simulink library "Golf_Components_Lib"  (R2018a)
settings: Solver=ode45  StartTime=0.0  StopTime=10.0  RelTol=1e-3  EnableMultiTasking=on
undefined symbols (not defined in the file): Plane_Data_Ring, X, Y, Z
libraries: sm_lib x63, Contact_Forces_Lib x21, nesl_utility x4
(part 1 of 3)
Description:
  | Copyright 2015-2019 The MathWorks, Inc.
settings Model: Creator=smiller  LastModifiedBy=smiller
settings DataIOCC: LimitDataPoints=on  SaveFormat=Array  SignalLoggingSaveFormat=ModelDataLogs
settings OptimizationCC: ExpressionDepthLimit=2147483647  LifeSpan=inf
settings DebuggingCC: UnderspecifiedInitializationDetection=Classic  MergeDetectMultiDrivingBlocksExec=none  SolverPrmCheckMsg=warning  FcnCallInpInsideContextMsg=warning  AllowSymbolicDim=off  StateNameClashWarn=warning  SFUnexpectedBacktrackingDiag=warning  SFNoUnconditionalDefaultTransitionDiag=warning  SFExecutionAtInitializationDiag=none
settings HardwareCC: ProdBitPerPointer=32  ProdBitPerSizeT=32  ProdBitPerPtrDiffT=32  ProdLargestAtomicFloat=None  ProdIntDivRoundTo=Undefined  ProdEndianess=Unspecified  ProdWordSize=32  ProdHWDeviceType=32-bit Generic
settings ModelReferenceCC: PropagateSignalLabelsOutOfModel=off
settings CodeAppCC: StateflowObjectComments=on
settings GRTTargetCC: TargetLangStandard=C89/C90 (ANSI)  GeneratePreprocessorConditionals=Disable all
settings ConfigComp: CovMetricSettings=dw  CovHtmlReporting=on  CovSaveCumulativeToWorkspaceVar=on  CovSaveSingleToWorkspaceVar=on  CovExternalEMLEnable=off  CovSFcnEnable=off

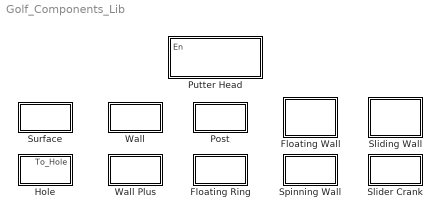
== system Golf_Components_Lib ==
  Floating Ring : Subsystem  mask(Floating Ring, 2D Contacts){extr_xy_data=Plane_Data_Ring(0.5,0.4), offset=[5.7 0 0], height=0.0853, diameter=0.5, extr1_friction=0.3, ball_radius=0.04267, contact_k=1e5, contact_b=10, low_pass_filt_const=1e-4}
      mask prompts: extr_xy_data "Extrusion XY Data (m)"; offset "Offset (x,y,z)"; diameter "Outer Diameter (m)"; extr1_friction "Friction (N/(m/s))"; ball_radius "Ball Radius (m)"; contact_k "Contact Stiffness"; contact_b "Contact Damping"; low_pass_filt_const "Low Pass Filter Constant"
      mask help:
      | Parameterized ring with integrated contact forces that will repel a circle.  The ring can translate only within the XY plane.
      |
      | The port must be connected to a frame located at the center of a circle.  The Ref Frame should be connected to the World Frame.
  Floating Wall : Subsystem  mask(Floating Wall with Round Ends, 2D Contacts){length=1.8, angle=0, offset=[5 0 0], height=0.0853, width=0.1, wall_friction=0.3, wall_rot_friction=0.1, ball_radius=0.04267, contact_k=1e5, contact_b=10, low_pass_filt_const=1e-4}
      mask prompts: length "Length (m)"; angle "Angle (deg)"; offset "Offset (x,y,z)"; wall_friction "Wall Sliding Friction(N/(m/s))"; wall_rot_friction "Wall Spinning Friction(N*m/(rad/s))"; ball_radius "Ball Radius (m)"; contact_k "Contact Stiffness"; contact_b "Contact Damping"; low_pass_filt_const "Low Pass Filter Constant"
      mask help:
      | Parameterized wall section with round ends with integrated contact forces that will repel a circle.  The wall can translate and rotate within the XY-plane.
      |
      | The Ball port must be connected to a frame located at the center of a circle. The Ref port should be connected to the World Frame. The C1 and C2 ports are connected to frames at the centers of the circles at either end of the wall.  Connecting these to Circle-to-Plane forces will enable the wall to bounce off of other walls.
  Hole : Subsystem  mask(Golf Course Hole, with Attractor Force){hole_offset=[5.5  0   -0.05], hole_radius=0.1079, hole_height=0.0505, hole_stiffness=-1e4, hole_damping=10, hole_deadzone=0.6667}
      mask prompts: hole_offset "Hole Location (x,y,z)"; hole_radius "Hole Radius (m)"; hole_height "Hole Height(m)"; hole_stiffness "Hole Attraction Stiffness"; hole_damping "Hole Attraction Damping"; hole_deadzone "Hole Deadzone (m)/Hole Radius (m)"
      mask help: Creates a hole for the golf course. The circle-to-circle attraction force will draw the ball into the hole if it gets close enough. The deadzone at the center of the hole is to reduce oscillations when the ball arrives. Outputs are the distance from the ball to the hole (x, y, r, and theta).
      mask DialogControl ParameterTabVar0 Prompt: Location
      mask DialogControl ParameterTabVar01 Prompt: Dimensions
      mask DialogControl ParameterTabVar012 Prompt: Contact
  Post : Subsystem  mask(Round Obstacle, 2D Contacts){width=1.2, height=0.0853, offset=[2.2 -0.25 0], ball_radius=0.04267, contact_k=1e5, contact_b=10, low_pass_filt_const=1e-4}
      mask prompts: width "Diameter (m)"; height "Height (m)"; offset "Offset (x,y,z)"; ball_radius "Ball Radius (m)"; contact_k "Contact Stiffness"; contact_b "Contact Damping"; low_pass_filt_const "Low Pass Filter Constant"
      mask help:
      | Parameterized round obstacle with integrated contact forces that will repel a circle.
      |
      | The Ball port must be connected to a frame located at the center of a circle.  The Ref port should be connected to a World Frame.
  Putter Head : Subsystem  mask(Wall with Round Ends, 2D Contact Forces){length=0.1270, height=0.03, width=0.05, ball_radius=0.04267, contact_k=1e5, contact_b=10, low_pass_filt_const=1e-4}
      mask prompts: length "Length (m)"; ball_radius "Ball Radius (m)"; contact_k "Contact Stiffness"; contact_b "Contact Damping"; low_pass_filt_const "Low Pass Filter Constant"
      mask help: Parameterized wall section with round ends with integrated contact forces that will repel a circle. The port must be connected to a frame located at the center of a circle.
      mask Display:
      | image(imread('Putter_Head_IMAGE.jpg'));
      | port_label('input',1,'En');
      | port_label('LConn',1,'CG');
      | port_label('RConn',1,'Ball');
  Slider Crank : Subsystem  mask(Slider Crank){initial_crank_spd=1, initial_crank_ang=0, rod_pin_radius=0.01, rod_pin_length=0.15, rod_pin_z_offset=-0.05, rod_dims=[0.025 0.75 0.015], rod_z_offset=-0.05, crank_pin_radius=0.01, crank_pin_length=0.05, crank_radius=0.25, crank_length=0.05, crank_z_offset=-0.05, density=1000}
      mask prompts: initial_crank_spd "Initial Crank Speed (rad/s)"; initial_crank_ang "Initial Crank Angle (deg)"; rod_pin_radius "Rod Pin Radius (m)"; rod_pin_length "Rod Pin Length (m)"; rod_pin_z_offset "Rod Pin Z Offset (m)"; rod_dims "Rod Dimensions (m)"; rod_z_offset "Rod Z Offset (m)"; crank_pin_radius "Crank Pin Radius (m)"; crank_pin_length "Crank Pin Length (m)"; crank_radius "Crank Radius (m)"; crank_length "Crank_Length (m)"; crank_z_offset "Crank Z Offset (m)"; density "Part Density (kg/m^3)"
      mask help:
      | Crank, sliding rod, and pin for connection to a slider.
      |
      | FRodPin should be connected to the part representing the slider.  FCrankCG should be attached to the World Frame at the same location as FRodPin.  Mechanism is parameterized relative to the slider pin location.
  Sliding Wall : Subsystem  mask(Sliding Wall with Round Ends, 2D Contacts){length=2, angle=0, offset=[1.5 -0.5 0], height=0.0853, width=0.1, wall_density=1000, ball_radius=0.0427, contact_k=1e5, contact_b=10, low_pass_filt_const=1e-4}
      mask prompts: length "Length (m)"; angle "Angle (deg)"; offset "Offset (x,y,z)"; wall_density "Wall Density (kg/m3)"; ball_radius "Ball Radius (m)"; contact_k "Contact Stiffness"; contact_b "Contact Damping"; low_pass_filt_const "Low Pass Filter Constant"
      mask help:
      | Parameterized wall section with round ends with integrated contact forces that will repel a circle.  This wall can slide along the Y axis only.
      |
      | The port must be connected to a frame located at the center of a circle. The Ref port should be connected to the World Frame.
      |
      | The WRf port is attached to the same part as Ref, and located at the center of the Offset position of the wall.  The Wall port is attached to the Wall CG, and is where the actuation for sliding can be attached.
  Spinning Wall : Subsystem  mask(Spinning Wall with Round Ends, 2D Contacts){length=1.8, angle=0, offset=[4 0 0], ang_spd=1, height=0.0853, width=0.1, wall_density=1000, ball_radius=0.0427, contact_k=1e5, contact_b=10, low_pass_filt_const=1e-4}
      mask prompts: length "Length (m)"; angle "Angle (deg)"; offset "Offset (x,y,z)"; ang_spd "Initial Speed (rad/s)"; wall_density "Wall Density (kg/m3)"; ball_radius "Ball Radius (m)"; contact_k "Contact Stiffness"; contact_b "Contact Damping"; low_pass_filt_const "Low Pass Filter Constant"
      mask help:
      | Parameterized wall section with round ends with integrated contact forces that will repel a circle.  This wall can rotate only within the XY plane.
      |
      | The port must be connected to a frame located at the center of a circle. The Ref port should be connected to the World Frame. Additional wall sections that will also rotate may be connected to the CG port.
  Surface : Subsystem  mask(Square Surface Patch for Golf Course){width=2, length=6, offset=[3 0 -0.05], height=0.05}
      mask prompts: width "Surface Width (m)"; length "Surface Length (m)"; offset "Surface Offset (m)"; height "Surface Thickness(m)"
      mask help: Creates a square surface patch for golf course. All parameters are relative to the frame that is connected to the port.
  Wall : Subsystem  mask(Wall with Round Ends, 2D Contacts){length=2, angle=0, offset=[6 0 0], height=0.0853, width=0.1, wall_density=1000, ball_radius=0.0427, contact_k=1e5, contact_b=10, low_pass_filt_const=1e-4}
      mask prompts: length "Length (m)"; angle "Angle (deg)"; offset "Offset (x,y,z)"; wall_density "Wall Density (kg/m3)"; ball_radius "Ball Radius (m)"; contact_k "Contact Stiffness"; contact_b "Contact Damping"; low_pass_filt_const "Low Pass Filter Constant"
      mask help: Parameterized wall section with round ends with integrated contact forces that will repel a circle. The Ball port must be connected to a frame located at the center of a circle. The Ref port should be connected to a World Frame
  Wall Plus : Subsystem  mask(Wall with Round Ends, 2D Contacts, Port at CG){length=2, angle=0, offset=[6 0 0], height=0.0853, width=0.1, ball_radius=0.04267, contact_k=1e5, contact_b=10, low_pass_filt_const=1e-4}
      mask prompts: length "Length (m)"; angle "Angle (deg)"; offset "Offset (x,y,z)"; ball_radius "Ball Radius (m)"; contact_k "Contact Stiffness"; contact_b "Contact Damping"; low_pass_filt_const "Low Pass Filter Constant"
      mask help: Parameterized wall section with round ends with integrated contact forces that will repel a circle. The Ball port must be connected to a frame located at the center of a circle. The Ref port should be connected to the World Frame. The Pla port can be used for addding additional contact forces.

== system Golf_Components_Lib/Floating Ring ==
  2-D Contact Force Circle to Circle1 : Contact_Forces_Lib/2D/Circle to Circle Force  cirB_rad=diameter/2  cirF_rad=ball_radius  active_angle=[-180 180]  force_law=Linear  k_contact=contact_k  b_contact=contact_b  pen_full_damp_F=1e-4  pen_exponent=1  custom_param_1=1  custom_param_2=1  friction_law=None  mu_kinetic=0.5  mu_static=0.7  v_thr=0.001  vis_on=off  vis_opc_en=0  vis_len_cirBz=0.1  vis_len_cirBx=0.005  vis_len_cirFz=0.1  vis_len_cirFx=0.005  vis_clr=[0.9 0.2 0.2]  vis_opc=0.7
      settings: SourceProductName=Simscape Multibody Contact Forces Library
  Offset and Angle : sm_lib/Frames and Transforms/Rigid Transform  TranslationMethod=Cartesian  TranslationStandardOffset=0  TranslationLengthUnit=m  TranslationStandardAxis=+Y  TranslationCartesianOffset=offset  TranslationROffset=0  TranslationROffsetUnits=m  TranslationZOffset=0  TranslationZOffsetUnits=m  TranslationThetaOffset=0  TranslationThetaOffsetUnits=deg  RotationMethod=None  RotationAngleUnits=deg  RotationStandardAxis=+Z  RotationAngle=0  RotationArbitraryAxis=[0 0 1]  FollAlignAxisA=+X  BaseAlignAxisA=+Y  FollAlignAxisB=+Y  BaseAlignAxisB=+Z  RotationSequenceAxes=FollowerAxes  RotationSequence=XYX  RotationSequenceAngles=[0 0 0]  RotationSequenceAnglesUnits=deg  RotationMatrix=[1 0 0; 0 1 0; 0 0 1]
  Rectangular Joint : sm_lib/Joints/Rectangular Joint  SenseConstraintForce=off  SenseConstraintForceX=off  SenseConstraintForceY=off  SenseConstraintForceZ=off  SenseConstraintTorque=off  SenseConstraintTorqueX=off  SenseConstraintTorqueY=off  SenseConstraintTorqueZ=off  SenseTotalForce=off  SenseTotalForceX=off  SenseTotalForceY=off  SenseTotalForceZ=off  SenseTotalTorque=off  SenseTotalTorqueX=off  SenseTotalTorqueY=off  SenseTotalTorqueZ=off  CompositeWrenchDir=FollowerOnBase  CompositeWrenchFrame=BaseFrame  PxEquilibriumPosition=0  PxEquilibriumPositionUnits=m  PxSpringStiffness=0  PxSpringStiffnessUnits=N/m  PxDampingCoefficient=extr1_friction  PxDampingCoefficientUnits=N/(m/s)  PxTorqueActuationMode=NoTorque  PxMotionActuationMode=ComputedMotion  PxSensePosition=off  PxSenseVelocity=off  PxSenseAcceleration=off  PxSenseTorqueForce=off  PxPositionTargetSpecify=off  PxPositionTargetPriority=High  PxPositionTargetValue=0  PxPositionTargetValueUnits=m  PxVelocityTargetSpecify=off  PxVelocityTargetPriority=High  PxVelocityTargetValue=0  PxVelocityTargetValueUnits=m/s  PyEquilibriumPosition=0  PyEquilibriumPositionUnits=m  PySpringStiffness=0  PySpringStiffnessUnits=N/m  PyDampingCoefficient=extr1_friction  PyDampingCoefficientUnits=N/(m/s)  PyTorqueActuationMode=NoTorque  PyMotionActuationMode=ComputedMotion  PySensePosition=off  PySenseVelocity=off  PySenseAcceleration=off  PySenseTorqueForce=off  PyPositionTargetSpecify=off  PyPositionTargetPriority=High  PyPositionTargetValue=0  PyPositionTargetValueUnits=m  PyVelocityTargetSpecify=off  PyVelocityTargetPriority=High  PyVelocityTargetValue=0  PyVelocityTargetValueUnits=m/s
      settings: SourceProductName=Simscape Multibody
  Ring : sm_lib/Body Elements/Solid  InertiaType=CalculateFromGeometry  Mass=1  MassUnits=kg  CenterOfMass=[0 0 0]  CenterOfMassUnits=m  MomentsOfInertia=[1 1 1]  MomentsOfInertiaUnits=kg*m^2  ProductsOfInertia=[0 0 0]  ProductsOfInertiaUnits=kg*m^2  DensityBased=on  Density=Mini_Golf_Param.Hole_7.Wall_Obst1.Density  DensityUnits=kg/(m^3)  DoExposeReferenceFrame=on  SerializedFrames=<Frames/>  GraphicType=FromGeometry  MarkerShape=Sphere  MarkerSize=10  MarkerSizeUnits=m  GraphicVisPropType=SimpleVisualProperties  GraphicDiffuseColor=[0.5 0.5 0.5]  GraphicSpecularColor=[0.5 0.5 0.5 1.0]  GraphicAmbientColor=[0.15 0.15 0.15 1.0]  GraphicEmissiveColor=[0.0 0.0 0.0 1.0]  GraphicShininess=75  GraphicOpacity=1.0  GeometryShape=GeneralExtrusion  RectangleSize=[1 1]  RectangleSizeUnits=m  BrickDimensions=[1 1 1]  BrickDimensionUnits=m  CylinderRadius=1  CylinderRadiusUnits=m  CylinderLength=1  CylinderLengthUnits=m  SphereRadius=1  SphereRadiusUnits=m  EllipsoidRadii=[1 1 1]  EllipsoidRadiiUnits=m  ExtrusionCrossSection=extr_xy_data  ExtrusionCrossSectionUnits=m  ExtrusionLength=height  ExtrusionLengthUnits=m  PolygonNumSides=3  PolygonOuterRadius=1  PolygonOuterRadiusUnits=m  ExtGeomFileType=STL  ExtGeomFileUnits=m  RevolutionCrossSection=[1 1; 1 -1; 2 -1; 2 1]  RevolutionCrossSectionUnits=m  RevolutionExtent=Full  RevolutionAngle=180  RevolutionAngleUnits=deg
  Terminator : Terminator
  Ball : PMIOPort  Side=Right
  Ref : PMIOPort  Port=2  Side=Left
  CG : PMIOPort  Port=3  Side=Left
  wires:
  2-D Contact Force Circle to Circle1/1 -> Terminator/1
  connections:
  Offset and Angle/LConn1 -- Ref/RConn1
  Offset and Angle/RConn1 -- Rectangular Joint/RConn1
  2-D Contact Force Circle to Circle1/RConn1 -- CG/RConn1 -- Rectangular Joint/LConn1 -- Ring/RConn1
  2-D Contact Force Circle to Circle1/LConn1 -- Ball/RConn1

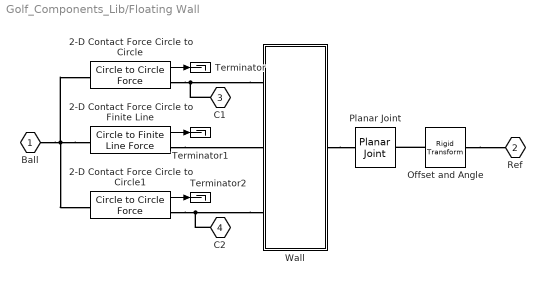
== system Golf_Components_Lib/Floating Wall ==
  2-D Contact Force Circle to Circle : Contact_Forces_Lib/2D/Circle to Circle Force  cirB_rad=width/2  cirF_rad=ball_radius  active_angle=[-180 180]  force_law=Linear  k_contact=contact_k  b_contact=contact_b  pen_full_damp_F=1e-4  pen_exponent=1  custom_param_1=1  custom_param_2=1  friction_law=None  mu_kinetic=0.5  mu_static=0.7  v_thr=0.001  vis_on=off  vis_opc_en=0  vis_len_cirBz=0.1  vis_len_cirBx=0.005  vis_len_cirFz=0.1  vis_len_cirFx=0.005  vis_clr=[0.9 0.2 0.2]  vis_opc=0.7
      settings: SourceProductName=Simscape Multibody Contact Forces Library
  2-D Contact Force Circle to Circle1 : Contact_Forces_Lib/2D/Circle to Circle Force  cirB_rad=width/2  cirF_rad=ball_radius  active_angle=[-180 180]  force_law=Linear  k_contact=contact_k  b_contact=contact_b  pen_full_damp_F=1e-4  pen_exponent=1  custom_param_1=1  custom_param_2=1  friction_law=None  mu_kinetic=0.5  mu_static=0.7  v_thr=0.001  vis_on=off  vis_opc_en=0  vis_len_cirBz=0.1  vis_len_cirBx=0.005  vis_len_cirFz=0.1  vis_len_cirFx=0.005  vis_clr=[0.9 0.2 0.2]  vis_opc=0.7
      settings: SourceProductName=Simscape Multibody Contact Forces Library
  2-D Contact Force Circle to Finite Line : Contact_Forces_Lib/2D/Circle to Finite Line Force  circle_rad=ball_radius  line_depth=width/2  line_length=length  force_law=Linear  k_contact=contact_k  b_contact=contact_b  pen_full_damp_F=1e-4  pen_exponent=1  custom_param_1=1  custom_param_2=1  friction_law=None  mu_kinetic=0.5  mu_static=0.7  v_thr=0.001  vis_on=off  vis_opc_en=0  vis_len_linBz=0.1  vis_len_linBx=0.005  vis_len_cirFz=0.1  vis_len_cirFx=0.005  vis_clr=[0.9 0.2 0.2]  vis_opc=0.7
      settings: SourceProductName=Simscape Multibody Contact Forces Library
  Offset and Angle : sm_lib/Frames and Transforms/Rigid Transform  TranslationMethod=Cartesian  TranslationStandardOffset=length/2  TranslationLengthUnit=m  TranslationStandardAxis=+Y  TranslationCartesianOffset=offset  TranslationROffset=0  TranslationROffsetUnits=m  TranslationZOffset=0  TranslationZOffsetUnits=m  TranslationThetaOffset=0  TranslationThetaOffsetUnits=deg  RotationMethod=StandardAxis  RotationAngleUnits=deg  RotationStandardAxis=+Z  RotationAngle=angle  RotationArbitraryAxis=[0 0 1]  FollAlignAxisA=+X  BaseAlignAxisA=+Y  FollAlignAxisB=+Y  BaseAlignAxisB=+Z  RotationSequenceAxes=FollowerAxes  RotationSequence=XYX  RotationSequenceAngles=[0 0 0]  RotationSequenceAnglesUnits=deg  RotationMatrix=[1 0 0; 0 1 0; 0 0 1]
  Planar Joint : sm_lib/Joints/Planar Joint  SenseConstraintForce=off  SenseConstraintForceX=off  SenseConstraintForceY=off  SenseConstraintForceZ=off  SenseConstraintTorque=off  SenseConstraintTorqueX=off  SenseConstraintTorqueY=off  SenseConstraintTorqueZ=off  SenseTotalForce=off  SenseTotalForceX=off  SenseTotalForceY=off  SenseTotalForceZ=off  SenseTotalTorque=off  SenseTotalTorqueX=off  SenseTotalTorqueY=off  SenseTotalTorqueZ=off  CompositeWrenchDir=FollowerOnBase  CompositeWrenchFrame=BaseFrame  PxEquilibriumPosition=0  PxEquilibriumPositionUnits=m  PxSpringStiffness=0  PxSpringStiffnessUnits=N/m  PxDampingCoefficient=wall_friction  PxDampingCoefficientUnits=N/(m/s)  PxTorqueActuationMode=NoTorque  PxMotionActuationMode=ComputedMotion  PxSensePosition=off  PxSenseVelocity=off  PxSenseAcceleration=off  PxSenseTorqueForce=off  PxPositionTargetSpecify=off  PxPositionTargetPriority=High  PxPositionTargetValue=0  PxPositionTargetValueUnits=m  PxVelocityTargetSpecify=off  PxVelocityTargetPriority=High  PxVelocityTargetValue=0  PxVelocityTargetValueUnits=m/s  PyEquilibriumPosition=0  PyEquilibriumPositionUnits=m  PySpringStiffness=0  PySpringStiffnessUnits=N/m  PyDampingCoefficient=wall_friction  PyDampingCoefficientUnits=N/(m/s)  PyTorqueActuationMode=NoTorque  PyMotionActuationMode=ComputedMotion  PySensePosition=off  PySenseVelocity=off  PySenseAcceleration=off  PySenseTorqueForce=off  PyPositionTargetSpecify=off  PyPositionTargetPriority=High  PyPositionTargetValue=0  PyPositionTargetValueUnits=m  PyVelocityTargetSpecify=off  PyVelocityTargetPriority=High  PyVelocityTargetValue=0  PyVelocityTargetValueUnits=m/s  RzEquilibriumPosition=0  RzEquilibriumPositionUnits=rad  RzSpringStiffness=0  RzSpringStiffnessUnits=N*m/rad  RzDampingCoefficient=wall_rot_friction  RzDampingCoefficientUnits=N*m/(rad/s)  RzTorqueActuationMode=NoTorque  RzMotionActuationMode=ComputedMotion  RzSensePosition=off  RzSenseVelocity=off  RzSenseAcceleration=off  RzSenseTorqueForce=off  RzPositionTargetSpecify=off  RzPositionTargetPriority=High  RzPositionTargetValue=0  RzPositionTargetValueUnits=rad  RzVelocityTargetSpecify=off  RzVelocityTargetPriority=High  RzVelocityTargetValue=0  RzVelocityTargetValueUnits=rad/s
  Terminator : Terminator
  Terminator1 : Terminator
  Terminator2 : Terminator
  Wall : Subsystem
  Ball : PMIOPort  Side=Right
  Ref : PMIOPort  Port=2  Side=Left
  C1 : PMIOPort  Port=3  Side=Left
  C2 : PMIOPort  Port=4  Side=Left
  wires:
  2-D Contact Force Circle to Circle/1 -> Terminator/1
  2-D Contact Force Circle to Finite Line/1 -> Terminator1/1
  2-D Contact Force Circle to Circle1/1 -> Terminator2/1
  connections:
  2-D Contact Force Circle to Finite Line/LConn1 -- 2-D Contact Force Circle to Circle1/LConn1 -- Ball/RConn1 -- 2-D Contact Force Circle to Circle/LConn1
  Offset and Angle/RConn1 -- Planar Joint/LConn1
  Offset and Angle/LConn1 -- Ref/RConn1
  Wall/RConn1 -- C1/RConn1 -- 2-D Contact Force Circle to Circle/RConn1
  2-D Contact Force Circle to Finite Line/RConn1 -- Wall/RConn2
  Wall/LConn1 -- Planar Joint/RConn1
  Wall/RConn3 -- C2/RConn1 -- 2-D Contact Force Circle to Circle1/RConn1

== system Golf_Components_Lib/Hole ==
  2-D Attraction Force Circle to Hole : Contact_Forces_Lib/2D/Circle to Hole Force  k_contact=hole_stiffness  b_contact=hole_damping  max_frame_sep=hole_radius  active_angle=[-180 180]  h_deadzone=hole_deadzone
      settings: SourceProductName=Simscape Multibody Contact Forces Library
  Hole : sm_lib/Body Elements/Solid  InertiaType=CalculateFromGeometry  Mass=1  MassUnits=kg  CenterOfMass=[0 0 0]  CenterOfMassUnits=m  MomentsOfInertia=[1 1 1]  MomentsOfInertiaUnits=kg*m^2  ProductsOfInertia=[0 0 0]  ProductsOfInertiaUnits=kg*m^2  DensityBased=on  Density=100  DensityUnits=kg/(m^3)  DoExposeReferenceFrame=on  SerializedFrames=<Frames/>  GraphicType=FromGeometry  MarkerShape=Sphere  MarkerSize=10  MarkerSizeUnits=m  GraphicVisPropType=SimpleVisualProperties  GraphicDiffuseColor=[0.0 0.0 0.0]  GraphicSpecularColor=[0.5 0.5 0.5 1.0]  GraphicAmbientColor=[0.15 0.15 0.15 1.0]  GraphicEmissiveColor=[0.0 0.0 0.0 1.0]  GraphicShininess=75  GraphicOpacity=1.0  GeometryShape=Cylinder  RectangleSize=[1 1]  RectangleSizeUnits=m  BrickDimensions=[1 1 1]  BrickDimensionUnits=m  CylinderRadius=hole_radius  CylinderRadiusUnits=m  CylinderLength=hole_height  CylinderLengthUnits=m  SphereRadius=1  SphereRadiusUnits=m  EllipsoidRadii=[1 1 1]  EllipsoidRadiiUnits=m  ExtrusionCrossSection=[1 1; -1 1; -1 -1; 1 -1]  ExtrusionCrossSectionUnits=m  ExtrusionLength=1  ExtrusionLengthUnits=m  PolygonNumSides=3  PolygonOuterRadius=1  PolygonOuterRadiusUnits=m  ExtGeomFileType=STL  ExtGeomFileUnits=m  RevolutionCrossSection=[1 1; 1 -1; 2 -1; 2 1]  RevolutionCrossSectionUnits=m  RevolutionExtent=Full  RevolutionAngle=180  RevolutionAngleUnits=deg
  Rigid Transform : sm_lib/Frames and Transforms/Rigid Transform  TranslationMethod=Cartesian  TranslationStandardOffset=0  TranslationLengthUnit=m  TranslationStandardAxis=+Z  TranslationCartesianOffset=hole_offset  TranslationROffset=0  TranslationROffsetUnits=m  TranslationZOffset=0  TranslationZOffsetUnits=m  TranslationThetaOffset=0  TranslationThetaOffsetUnits=deg  RotationMethod=None  RotationAngleUnits=deg  RotationStandardAxis=+Z  RotationAngle=0  RotationArbitraryAxis=[0 0 1]  FollAlignAxisA=+X  BaseAlignAxisA=+Y  FollAlignAxisB=+Y  BaseAlignAxisB=+Z  RotationSequenceAxes=FollowerAxes  RotationSequence=XYX  RotationSequenceAngles=[0 0 0]  RotationSequenceAnglesUnits=deg  RotationMatrix=[1 0 0; 0 1 0; 0 0 1]
  Sensing : Subsystem
  Terminator : Terminator
  Ball : PMIOPort  Side=Left
  Ref : PMIOPort  Port=2  Side=Right
  To_Hole : Outport
  wires:
  Sensing/1(To_Hole) -> To_Hole/1
  2-D Attraction Force Circle to Hole/1 -> Terminator/1
  connections:
  Rigid Transform/LConn1 -- Ref/RConn1
  Hole/RConn1 -- Rigid Transform/RConn1 -- Sensing/RConn1 -- 2-D Attraction Force Circle to Hole/RConn1
  Sensing/LConn1 -- Ball/RConn1 -- 2-D Attraction Force Circle to Hole/LConn1

== system Golf_Components_Lib/Post ==
  2-D Contact Force Circle to Circle : Contact_Forces_Lib/2D/Circle to Circle Force  cirB_rad=width/2  cirF_rad=ball_radius  active_angle=[-180 180]  force_law=Linear  k_contact=contact_k  b_contact=contact_b  pen_full_damp_F=1e-4  pen_exponent=1  custom_param_1=1  custom_param_2=1  friction_law=None  mu_kinetic=0.5  mu_static=0.7  v_thr=0.001  vis_on=off  vis_opc_en=0  vis_len_cirBz=0.1  vis_len_cirBx=0.005  vis_len_cirFz=0.1  vis_len_cirFx=0.005  vis_clr=[0.9 0.2 0.2]  vis_opc=0.7
      settings: SourceProductName=Simscape Multibody Contact Forces Library
  Offset and Angle : sm_lib/Frames and Transforms/Rigid Transform  TranslationMethod=Cartesian  TranslationStandardOffset=0  TranslationLengthUnit=m  TranslationStandardAxis=+Y  TranslationCartesianOffset=offset  TranslationROffset=0  TranslationROffsetUnits=m  TranslationZOffset=0  TranslationZOffsetUnits=m  TranslationThetaOffset=0  TranslationThetaOffsetUnits=deg  RotationMethod=None  RotationAngleUnits=deg  RotationStandardAxis=+Z  RotationAngle=0  RotationArbitraryAxis=[0 0 1]  FollAlignAxisA=+X  BaseAlignAxisA=+Y  FollAlignAxisB=+Y  BaseAlignAxisB=+Z  RotationSequenceAxes=FollowerAxes  RotationSequence=XYX  RotationSequenceAngles=[0 0 0]  RotationSequenceAnglesUnits=deg  RotationMatrix=[1 0 0; 0 1 0; 0 0 1]
  Post : sm_lib/Body Elements/Solid  InertiaType=CalculateFromGeometry  Mass=1  MassUnits=kg  CenterOfMass=[0 0 0]  CenterOfMassUnits=m  MomentsOfInertia=[1 1 1]  MomentsOfInertiaUnits=kg*m^2  ProductsOfInertia=[0 0 0]  ProductsOfInertiaUnits=kg*m^2  DensityBased=on  Density=1  DensityUnits=kg/(m^3)  DoExposeReferenceFrame=on  SerializedFrames=<Frames/>  GraphicType=FromGeometry  MarkerShape=Sphere  MarkerSize=10  MarkerSizeUnits=m  GraphicVisPropType=SimpleVisualProperties  GraphicDiffuseColor=[0.5 0.5 0.5]  GraphicSpecularColor=[0.5 0.5 0.5 1.0]  GraphicAmbientColor=[0.15 0.15 0.15 1.0]  GraphicEmissiveColor=[0.0 0.0 0.0 1.0]  GraphicShininess=75  GraphicOpacity=1.0  GeometryShape=Cylinder  RectangleSize=[1 1]  RectangleSizeUnits=m  BrickDimensions=[1 1 1]  BrickDimensionUnits=m  CylinderRadius=width/2  CylinderRadiusUnits=m  CylinderLength=height  CylinderLengthUnits=m  SphereRadius=1  SphereRadiusUnits=m  EllipsoidRadii=[1 1 1]  EllipsoidRadiiUnits=m  ExtrusionCrossSection=[1 1; -1 1; -1 -1; 1 -1]  ExtrusionCrossSectionUnits=m  ExtrusionLength=1  ExtrusionLengthUnits=m  PolygonNumSides=3  PolygonOuterRadius=1  PolygonOuterRadiusUnits=m  ExtGeomFileType=STL  ExtGeomFileUnits=m  RevolutionCrossSection=[1 1; 1 -1; 2 -1; 2 1]  RevolutionCrossSectionUnits=m  RevolutionExtent=Full  RevolutionAngle=180  RevolutionAngleUnits=deg
  Terminator : Terminator
  Ball : PMIOPort  Side=Right
  Ref : PMIOPort  Port=2  Side=Left
  wires:
  2-D Contact Force Circle to Circle/1 -> Terminator/1
  connections:
  Ball/RConn1 -- 2-D Contact Force Circle to Circle/LConn1
  Offset and Angle/RConn1 -- 2-D Contact Force Circle to Circle/RConn1 -- Post/RConn1
  Offset and Angle/LConn1 -- Ref/RConn1

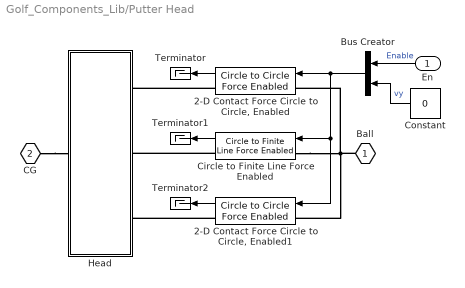
== system Golf_Components_Lib/Putter Head ==
  En : Inport
  "2-D Contact Force Circle to Circle, Enabled" : Contact_Forces_Lib/2D/Circle to Circle Force Enabled  cirB_rad=width/2  cirF_rad=ball_radius  active_angle=[-180 180]  force_law=Linear  k_contact=contact_k  b_contact=contact_b  pen_full_damp_F=1e-4  pen_exponent=1  custom_param_1=1  custom_param_2=1  friction_law=None  mu_kinetic=0.5  mu_static=0.7  v_thr=0.001  vis_on=off  vis_opc_en=0  vis_len_cirBz=0.1  vis_len_cirBx=0.005  vis_len_cirFz=0.1  vis_len_cirFx=0.005  vis_clr=[0.9 0.2 0.2]  vis_opc=0.7
      settings: SourceProductName=Simscape Multibody Contact Forces Library
  "2-D Contact Force Circle to Circle, Enabled1" : Contact_Forces_Lib/2D/Circle to Circle Force Enabled  cirB_rad=width/2  cirF_rad=ball_radius  active_angle=[-180 180]  force_law=Linear  k_contact=contact_k  b_contact=contact_b  pen_full_damp_F=1e-4  pen_exponent=1  custom_param_1=1  custom_param_2=1  friction_law=None  mu_kinetic=0.5  mu_static=0.7  v_thr=0.001  vis_on=off  vis_opc_en=0  vis_len_cirBz=0.1  vis_len_cirBx=0.005  vis_len_cirFz=0.1  vis_len_cirFx=0.005  vis_clr=[0.9 0.2 0.2]  vis_opc=0.7
      settings: SourceProductName=Simscape Multibody Contact Forces Library
  Bus Creator : BusCreator  Inputs=2
  Circle to Finite Line Force Enabled : Contact_Forces_Lib/2D/Circle to Finite Line Force Enabled  circle_rad=ball_radius  line_depth=width/2  line_length=length  force_law=Linear  k_contact=contact_k  b_contact=contact_b  pen_full_damp_F=1e-4  pen_exponent=1  custom_param_1=1  custom_param_2=1  friction_law=None  mu_kinetic=0.5  mu_static=0.7  v_thr=0.001  vis_on=off  vis_opc_en=0  vis_len_linBz=0.1  vis_len_linBx=0.005  vis_len_cirFz=0.1  vis_len_cirFx=0.005  vis_clr=[0.9 0.2 0.2]  vis_opc=0.7
      settings: SourceProductName=Simscape Multibody Contact Forces Library
  Constant : Constant  Value=0
  Head : Subsystem
  Terminator : Terminator
  Terminator1 : Terminator
  Terminator2 : Terminator
  Ball : PMIOPort  Side=Right
  CG : PMIOPort  Port=2  Side=Left
  wires:
  En/1 -> Bus Creator/1  "Enable"
  "2-D Contact Force Circle to Circle, Enabled"/1 -> Terminator/1
  Circle to Finite Line Force Enabled/1 -> Terminator1/1
  "2-D Contact Force Circle to Circle, Enabled1"/1 -> Terminator2/1
  Bus Creator/1 -> Circle to Finite Line Force Enabled/1, "2-D Contact Force Circle to Circle, Enabled1"/1, "2-D Contact Force Circle to Circle, Enabled"/1
  Constant/1 -> Bus Creator/2  "vy"
  connections:
  Ball/RConn1 -- Circle to Finite Line Force Enabled/LConn1 -- "2-D Contact Force Circle to Circle, Enabled"/LConn1 -- "2-D Contact Force Circle to Circle, Enabled1"/LConn1
  "2-D Contact Force Circle to Circle, Enabled"/RConn1 -- Head/RConn1
  Circle to Finite Line Force Enabled/RConn1 -- Head/RConn2
  CG/RConn1 -- Head/LConn1
  "2-D Contact Force Circle to Circle, Enabled1"/RConn1 -- Head/RConn3

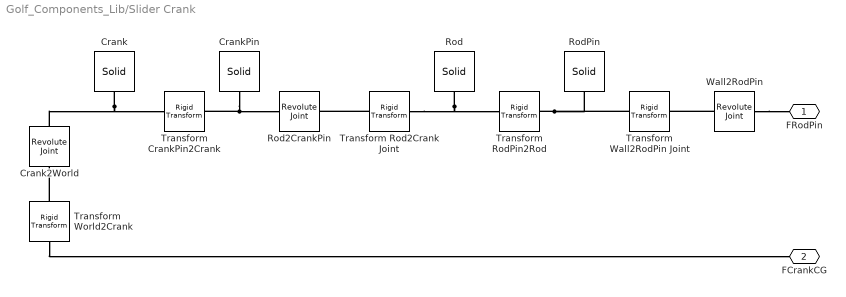
== system Golf_Components_Lib/Slider Crank ==
  Crank : sm_lib/Body Elements/Solid  InertiaType=CalculateFromGeometry  Mass=1  MassUnits=kg  CenterOfMass=[0 0 0]  CenterOfMassUnits=m  MomentsOfInertia=[1 1 1]  MomentsOfInertiaUnits=kg*m^2  ProductsOfInertia=[0 0 0]  ProductsOfInertiaUnits=kg*m^2  DensityBased=on  Density=density  DensityUnits=kg/(m^3)  DoExposeReferenceFrame=on  SerializedFrames=<Frames/>  GraphicType=FromGeometry  MarkerShape=Sphere  MarkerSize=10  MarkerSizeUnits=m  GraphicVisPropType=SimpleVisualProperties  GraphicDiffuseColor=[0.0 0.4 0.8]  GraphicSpecularColor=[0.5 0.5 0.5 1.0]  GraphicAmbientColor=[0.15 0.15 0.15 1.0]  GraphicEmissiveColor=[0.0 0.0 0.0 1.0]  GraphicShininess=75  GraphicOpacity=1.0  GeometryShape=Cylinder  RectangleSize=[1 1]  RectangleSizeUnits=m  BrickDimensions=[1 1 1]  BrickDimensionUnits=m  CylinderRadius=crank_radius  CylinderRadiusUnits=m  CylinderLength=crank_length  CylinderLengthUnits=m  SphereRadius=1  SphereRadiusUnits=m  EllipsoidRadii=[1 1 1]  EllipsoidRadiiUnits=m  ExtrusionCrossSection=[1 1; -1 1; -1 -1; 1 -1]  ExtrusionCrossSectionUnits=m  ExtrusionLength=1  ExtrusionLengthUnits=m  PolygonNumSides=3  PolygonOuterRadius=1  PolygonOuterRadiusUnits=m  ExtGeomFileType=STL  ExtGeomFileUnits=m  RevolutionCrossSection=[1 1; 1 -1; 2 -1; 2 1]  RevolutionCrossSectionUnits=m  RevolutionExtent=Full  RevolutionAngle=180  RevolutionAngleUnits=deg
  Crank2World : sm_lib/Joints/Revolute Joint  SenseConstraintForce=off  SenseConstraintForceX=off  SenseConstraintForceY=off  SenseConstraintForceZ=off  SenseConstraintTorque=off  SenseConstraintTorqueX=off  SenseConstraintTorqueY=off  SenseConstraintTorqueZ=off  SenseTotalForce=off  SenseTotalForceX=off  SenseTotalForceY=off  SenseTotalForceZ=off  SenseTotalTorque=off  SenseTotalTorqueX=off  SenseTotalTorqueY=off  SenseTotalTorqueZ=off  CompositeWrenchDir=FollowerOnBase  CompositeWrenchFrame=BaseFrame  EquilibriumPosition=0  EquilibriumPositionUnits=rad  SpringStiffness=0  SpringStiffnessUnits=N*m/rad  DampingCoefficient=0  DampingCoefficientUnits=N*m/(rad/s)  TorqueActuationMode=NoTorque  MotionActuationMode=ComputedMotion  SensePosition=off  SenseVelocity=off  SenseAcceleration=off  SenseTorqueForce=off  PositionTargetSpecify=on  PositionTargetPriority=High  PositionTargetValue=initial_crank_ang  PositionTargetValueUnits=deg  VelocityTargetSpecify=on  VelocityTargetPriority=High  VelocityTargetValue=initial_crank_spd  VelocityTargetValueUnits=rad/s
  CrankPin : sm_lib/Body Elements/Solid  InertiaType=CalculateFromGeometry  Mass=1  MassUnits=kg  CenterOfMass=[0 0 0]  CenterOfMassUnits=m  MomentsOfInertia=[1 1 1]  MomentsOfInertiaUnits=kg*m^2  ProductsOfInertia=[0 0 0]  ProductsOfInertiaUnits=kg*m^2  DensityBased=on  Density=density  DensityUnits=kg/(m^3)  DoExposeReferenceFrame=on  SerializedFrames=<Frames/>  GraphicType=FromGeometry  MarkerShape=Sphere  MarkerSize=10  MarkerSizeUnits=m  GraphicVisPropType=SimpleVisualProperties  GraphicDiffuseColor=[0.0 0.4 0.8]  GraphicSpecularColor=[0.5 0.5 0.5 1.0]  GraphicAmbientColor=[0.15 0.15 0.15 1.0]  GraphicEmissiveColor=[0.0 0.0 0.0 1.0]  GraphicShininess=75  GraphicOpacity=1.0  GeometryShape=Cylinder  RectangleSize=[1 1]  RectangleSizeUnits=m  BrickDimensions=[1 1 1]  BrickDimensionUnits=m  CylinderRadius=crank_pin_radius  CylinderRadiusUnits=m  CylinderLength=crank_pin_length  CylinderLengthUnits=m  SphereRadius=1  SphereRadiusUnits=m  EllipsoidRadii=[1 1 1]  EllipsoidRadiiUnits=m  ExtrusionCrossSection=[1 1; -1 1; -1 -1; 1 -1]  ExtrusionCrossSectionUnits=m  ExtrusionLength=1  ExtrusionLengthUnits=m  PolygonNumSides=3  PolygonOuterRadius=1  PolygonOuterRadiusUnits=m  ExtGeomFileType=STL  ExtGeomFileUnits=m  RevolutionCrossSection=[1 1; 1 -1; 2 -1; 2 1]  RevolutionCrossSectionUnits=m  RevolutionExtent=Full  RevolutionAngle=180  RevolutionAngleUnits=deg
  Rod : sm_lib/Body Elements/Solid  InertiaType=CalculateFromGeometry  Mass=1  MassUnits=kg  CenterOfMass=[0 0 0]  CenterOfMassUnits=m  MomentsOfInertia=[1 1 1]  MomentsOfInertiaUnits=kg*m^2  ProductsOfInertia=[0 0 0]  ProductsOfInertiaUnits=kg*m^2  DensityBased=on  Density=density  DensityUnits=kg/(m^3)  DoExposeReferenceFrame=on  SerializedFrames=<Frames/>  GraphicType=FromGeometry  MarkerShape=Sphere  MarkerSize=10  MarkerSizeUnits=m  GraphicVisPropType=SimpleVisualProperties  GraphicDiffuseColor=[1.0 0.2 0.2]  GraphicSpecularColor=[0.5 0.5 0.5 1.0]  GraphicAmbientColor=[0.15 0.15 0.15 1.0]  GraphicEmissiveColor=[0.0 0.0 0.0 1.0]  GraphicShininess=75  GraphicOpacity=1.0  GeometryShape=Brick  RectangleSize=[1 1]  RectangleSizeUnits=m  BrickDimensions=rod_dims  BrickDimensionUnits=m  CylinderRadius=0.01  CylinderRadiusUnits=m  CylinderLength=0.05  CylinderLengthUnits=m  SphereRadius=1  SphereRadiusUnits=m  EllipsoidRadii=[1 1 1]  EllipsoidRadiiUnits=m  ExtrusionCrossSection=[1 1; -1 1; -1 -1; 1 -1]  ExtrusionCrossSectionUnits=m  ExtrusionLength=1  ExtrusionLengthUnits=m  PolygonNumSides=3  PolygonOuterRadius=1  PolygonOuterRadiusUnits=m  ExtGeomFileType=STL  ExtGeomFileUnits=m  RevolutionCrossSection=[1 1; 1 -1; 2 -1; 2 1]  RevolutionCrossSectionUnits=m  RevolutionExtent=Full  RevolutionAngle=180  RevolutionAngleUnits=deg
  Rod2CrankPin : sm_lib/Joints/Revolute Joint  SenseConstraintForce=off  SenseConstraintForceX=off  SenseConstraintForceY=off  SenseConstraintForceZ=off  SenseConstraintTorque=off  SenseConstraintTorqueX=off  SenseConstraintTorqueY=off  SenseConstraintTorqueZ=off  SenseTotalForce=off  SenseTotalForceX=off  SenseTotalForceY=off  SenseTotalForceZ=off  SenseTotalTorque=off  SenseTotalTorqueX=off  SenseTotalTorqueY=off  SenseTotalTorqueZ=off  CompositeWrenchDir=FollowerOnBase  CompositeWrenchFrame=BaseFrame  EquilibriumPosition=0  EquilibriumPositionUnits=rad  SpringStiffness=0  SpringStiffnessUnits=N*m/rad  DampingCoefficient=0  DampingCoefficientUnits=N*m/(rad/s)  TorqueActuationMode=NoTorque  MotionActuationMode=ComputedMotion  SensePosition=off  SenseVelocity=off  SenseAcceleration=off  SenseTorqueForce=off  PositionTargetSpecify=off  PositionTargetPriority=High  PositionTargetValue=0  PositionTargetValueUnits=rad  VelocityTargetSpecify=off  VelocityTargetPriority=High  VelocityTargetValue=0  VelocityTargetValueUnits=rad/s
  RodPin : sm_lib/Body Elements/Solid  InertiaType=CalculateFromGeometry  Mass=1  MassUnits=kg  CenterOfMass=[0 0 0]  CenterOfMassUnits=m  MomentsOfInertia=[1 1 1]  MomentsOfInertiaUnits=kg*m^2  ProductsOfInertia=[0 0 0]  ProductsOfInertiaUnits=kg*m^2  DensityBased=on  Density=density  DensityUnits=kg/(m^3)  DoExposeReferenceFrame=on  SerializedFrames=<Frames/>  GraphicType=FromGeometry  MarkerShape=Sphere  MarkerSize=10  MarkerSizeUnits=m  GraphicVisPropType=SimpleVisualProperties  GraphicDiffuseColor=[0.0 0.0 0.0]  GraphicSpecularColor=[0.5 0.5 0.5 1.0]  GraphicAmbientColor=[0.15 0.15 0.15 1.0]  GraphicEmissiveColor=[0.0 0.0 0.0 1.0]  GraphicShininess=75  GraphicOpacity=1.0  GeometryShape=Cylinder  RectangleSize=[1 1]  RectangleSizeUnits=m  BrickDimensions=[1 1 1]  BrickDimensionUnits=m  CylinderRadius=rod_pin_radius  CylinderRadiusUnits=m  CylinderLength=rod_pin_length  CylinderLengthUnits=m  SphereRadius=1  SphereRadiusUnits=m  EllipsoidRadii=[1 1 1]  EllipsoidRadiiUnits=m  ExtrusionCrossSection=[1 1; -1 1; -1 -1; 1 -1]  ExtrusionCrossSectionUnits=m  ExtrusionLength=1  ExtrusionLengthUnits=m  PolygonNumSides=3  PolygonOuterRadius=1  PolygonOuterRadiusUnits=m  ExtGeomFileType=STL  ExtGeomFileUnits=m  RevolutionCrossSection=[1 1; 1 -1; 2 -1; 2 1]  RevolutionCrossSectionUnits=m  RevolutionExtent=Full  RevolutionAngle=180  RevolutionAngleUnits=deg
  Transform CrankPin2Crank : sm_lib/Frames and Transforms/Rigid Transform  TranslationMethod=Cartesian  TranslationStandardOffset=0.4  TranslationLengthUnit=m  TranslationStandardAxis=+Y  TranslationCartesianOffset=[0 crank_radius*0.8 crank_z_offset]  TranslationROffset=0  TranslationROffsetUnits=m  TranslationZOffset=0  TranslationZOffsetUnits=m  TranslationThetaOffset=0  TranslationThetaOffsetUnits=deg  RotationMethod=None  RotationAngleUnits=deg  RotationStandardAxis=+Z  RotationAngle=0  RotationArbitraryAxis=[0 0 1]  FollAlignAxisA=+X  BaseAlignAxisA=+Y  FollAlignAxisB=+Y  BaseAlignAxisB=+Z  RotationSequenceAxes=FollowerAxes  RotationSequence=XYX  RotationSequenceAngles=[0 0 0]  RotationSequenceAnglesUnits=deg  RotationMatrix=[1 0 0; 0 1 0; 0 0 1]
  Transform Rod2Crank Joint : sm_lib/Frames and Transforms/Rigid Transform  TranslationMethod=StandardAxis  TranslationStandardOffset=rod_dims(2)/2-0.025  TranslationLengthUnit=m  TranslationStandardAxis=+Y  TranslationCartesianOffset=[0 0 0]  TranslationROffset=0  TranslationROffsetUnits=m  TranslationZOffset=0  TranslationZOffsetUnits=m  TranslationThetaOffset=0  TranslationThetaOffsetUnits=deg  RotationMethod=None  RotationAngleUnits=deg  RotationStandardAxis=+Z  RotationAngle=0  RotationArbitraryAxis=[0 0 1]  FollAlignAxisA=+X  BaseAlignAxisA=+Y  FollAlignAxisB=+Y  BaseAlignAxisB=+Z  RotationSequenceAxes=FollowerAxes  RotationSequence=XYX  RotationSequenceAngles=[0 0 0]  RotationSequenceAnglesUnits=deg  RotationMatrix=[1 0 0; 0 1 0; 0 0 1]
  Transform RodPin2Rod : sm_lib/Frames and Transforms/Rigid Transform  TranslationMethod=Cartesian  TranslationStandardOffset=0.4  TranslationLengthUnit=m  TranslationStandardAxis=+Y  TranslationCartesianOffset=[0 rod_dims(2)/2-0.025 rod_z_offset]  TranslationROffset=0  TranslationROffsetUnits=m  TranslationZOffset=0  TranslationZOffsetUnits=m  TranslationThetaOffset=0  TranslationThetaOffsetUnits=deg  RotationMethod=None  RotationAngleUnits=deg  RotationStandardAxis=+Z  RotationAngle=0  RotationArbitraryAxis=[0 0 1]  FollAlignAxisA=+X  BaseAlignAxisA=+Y  FollAlignAxisB=+Y  BaseAlignAxisB=+Z  RotationSequenceAxes=FollowerAxes  RotationSequence=XYX  RotationSequenceAngles=[0 0 0]  RotationSequenceAnglesUnits=deg  RotationMatrix=[1 0 0; 0 1 0; 0 0 1]
  Transform Wall2RodPin Joint : sm_lib/Frames and Transforms/Rigid Transform  TranslationMethod=StandardAxis  TranslationStandardOffset=rod_pin_z_offset  TranslationLengthUnit=m  TranslationStandardAxis=+Z  TranslationCartesianOffset=[0 0 -0.05]  TranslationROffset=0  TranslationROffsetUnits=m  TranslationZOffset=0  TranslationZOffsetUnits=m  TranslationThetaOffset=0  TranslationThetaOffsetUnits=deg  RotationMethod=None  RotationAngleUnits=deg  RotationStandardAxis=+Z  RotationAngle=0  RotationArbitraryAxis=[0 0 1]  FollAlignAxisA=+X  BaseAlignAxisA=+Y  FollAlignAxisB=+Y  BaseAlignAxisB=+Z  RotationSequenceAxes=FollowerAxes  RotationSequence=XYX  RotationSequenceAngles=[0 0 0]  RotationSequenceAnglesUnits=deg  RotationMatrix=[1 0 0; 0 1 0; 0 0 1]
  Transform World2Crank : sm_lib/Frames and Transforms/Rigid Transform  TranslationMethod=Cartesian  TranslationStandardOffset=0.4  TranslationLengthUnit=m  TranslationStandardAxis=+Y  TranslationCartesianOffset=[0 rod_dims(2)-0.05+crank_radius rod_pin_z_offset+rod_z_offset+crank_z_offset]  TranslationROffset=0  TranslationROffsetUnits=m  TranslationZOffset=0  TranslationZOffsetUnits=m  TranslationThetaOffset=0  TranslationThetaOffsetUnits=deg  RotationMethod=None  RotationAngleUnits=deg  RotationStandardAxis=+Z  RotationAngle=0  RotationArbitraryAxis=[0 0 1]  FollAlignAxisA=+X  BaseAlignAxisA=+Y  FollAlignAxisB=+Y  BaseAlignAxisB=+Z  RotationSequenceAxes=FollowerAxes  RotationSequence=XYX  RotationSequenceAngles=[0 0 0]  RotationSequenceAnglesUnits=deg  RotationMatrix=[1 0 0; 0 1 0; 0 0 1]
  Wall2RodPin : sm_lib/Joints/Revolute Joint  SenseConstraintForce=off  SenseConstraintForceX=off  SenseConstraintForceY=off  SenseConstraintForceZ=off  SenseConstraintTorque=off  SenseConstraintTorqueX=off  SenseConstraintTorqueY=off  SenseConstraintTorqueZ=off  SenseTotalForce=off  SenseTotalForceX=off  SenseTotalForceY=off  SenseTotalForceZ=off  SenseTotalTorque=off  SenseTotalTorqueX=off  SenseTotalTorqueY=off  SenseTotalTorqueZ=off  CompositeWrenchDir=FollowerOnBase  CompositeWrenchFrame=BaseFrame  EquilibriumPosition=0  EquilibriumPositionUnits=rad  SpringStiffness=0  SpringStiffnessUnits=N*m/rad  DampingCoefficient=0  DampingCoefficientUnits=N*m/(rad/s)  TorqueActuationMode=NoTorque  MotionActuationMode=ComputedMotion  SensePosition=off  SenseVelocity=off  SenseAcceleration=off  SenseTorqueForce=off  PositionTargetSpecify=off  PositionTargetPriority=High  PositionTargetValue=0  PositionTargetValueUnits=rad  VelocityTargetSpecify=off  VelocityTargetPriority=High  VelocityTargetValue=0  VelocityTargetValueUnits=rad/s
  FRodPin : PMIOPort  Side=Right
  FCrankCG : PMIOPort  Port=2  Side=Right
  connections:
  Transform World2Crank/LConn1 -- FCrankCG/RConn1
  Transform World2Crank/RConn1 -- Crank2World/RConn1
  CrankPin/RConn1 -- Rod2CrankPin/RConn1 -- Transform CrankPin2Crank/LConn1
  Crank/RConn1 -- Transform CrankPin2Crank/RConn1 -- Crank2World/LConn1
  Transform Rod2Crank Joint/RConn1 -- Rod2CrankPin/LConn1
  Rod/RConn1 -- Transform RodPin2Rod/RConn1 -- Transform Rod2Crank Joint/LConn1
  Wall2RodPin/LConn1 -- FRodPin/RConn1
  Transform RodPin2Rod/LConn1 -- RodPin/RConn1 -- Transform Wall2RodPin Joint/RConn1
  Wall2RodPin/RConn1 -- Transform Wall2RodPin Joint/LConn1

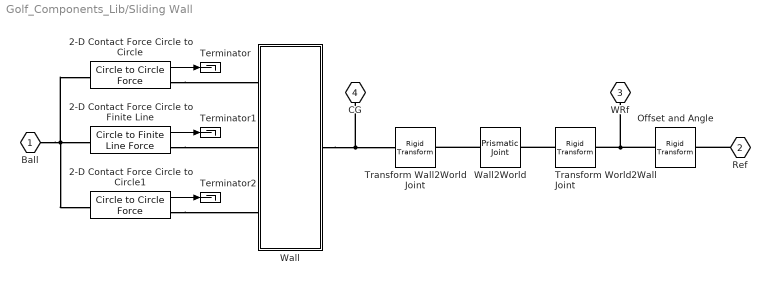
== system Golf_Components_Lib/Sliding Wall ==
  2-D Contact Force Circle to Circle : Contact_Forces_Lib/2D/Circle to Circle Force  cirB_rad=width/2  cirF_rad=ball_radius  active_angle=[-180 180]  force_law=Linear  k_contact=contact_k  b_contact=contact_b  pen_full_damp_F=1e-4  pen_exponent=1  custom_param_1=1  custom_param_2=1  friction_law=None  mu_kinetic=0.5  mu_static=0.7  v_thr=0.001  vis_on=off  vis_opc_en=0  vis_len_cirBz=0.1  vis_len_cirBx=0.005  vis_len_cirFz=0.1  vis_len_cirFx=0.005  vis_clr=[0.9 0.2 0.2]  vis_opc=0.7
      settings: SourceProductName=Simscape Multibody Contact Forces Library
  2-D Contact Force Circle to Circle1 : Contact_Forces_Lib/2D/Circle to Circle Force  cirB_rad=width/2  cirF_rad=ball_radius  active_angle=[-180 180]  force_law=Linear  k_contact=contact_k  b_contact=contact_b  pen_full_damp_F=1e-4  pen_exponent=1  custom_param_1=1  custom_param_2=1  friction_law=None  mu_kinetic=0.5  mu_static=0.7  v_thr=0.001  vis_on=off  vis_opc_en=0  vis_len_cirBz=0.1  vis_len_cirBx=0.005  vis_len_cirFz=0.1  vis_len_cirFx=0.005  vis_clr=[0.9 0.2 0.2]  vis_opc=0.7
      settings: SourceProductName=Simscape Multibody Contact Forces Library
  2-D Contact Force Circle to Finite Line : Contact_Forces_Lib/2D/Circle to Finite Line Force  circle_rad=ball_radius  line_depth=width/2  line_length=length  force_law=Linear  k_contact=contact_k  b_contact=contact_b  pen_full_damp_F=1e-4  pen_exponent=1  custom_param_1=1  custom_param_2=1  friction_law=None  mu_kinetic=0.5  mu_static=0.7  v_thr=0.001  vis_on=off  vis_opc_en=0  vis_len_linBz=0.1  vis_len_linBx=0.005  vis_len_cirFz=0.1  vis_len_cirFx=0.005  vis_clr=[0.9 0.2 0.2]  vis_opc=0.7
      settings: SourceProductName=Simscape Multibody Contact Forces Library
  Offset and Angle : sm_lib/Frames and Transforms/Rigid Transform  TranslationMethod=Cartesian  TranslationStandardOffset=0  TranslationLengthUnit=m  TranslationStandardAxis=+Y  TranslationCartesianOffset=offset  TranslationROffset=0  TranslationROffsetUnits=m  TranslationZOffset=0  TranslationZOffsetUnits=m  TranslationThetaOffset=0  TranslationThetaOffsetUnits=deg  RotationMethod=StandardAxis  RotationAngleUnits=deg  RotationStandardAxis=+Z  RotationAngle=angle  RotationArbitraryAxis=[0 0 1]  FollAlignAxisA=+X  BaseAlignAxisA=+Y  FollAlignAxisB=+Y  BaseAlignAxisB=+Z  RotationSequenceAxes=FollowerAxes  RotationSequence=XYX  RotationSequenceAngles=[0 0 0]  RotationSequenceAnglesUnits=deg  RotationMatrix=[1 0 0; 0 1 0; 0 0 1]
  Terminator : Terminator
  Terminator1 : Terminator
  Terminator2 : Terminator
  Transform Wall2World Joint : sm_lib/Frames and Transforms/Rigid Transform  TranslationMethod=Cartesian  TranslationStandardOffset=0.4  TranslationLengthUnit=m  TranslationStandardAxis=+Y  TranslationCartesianOffset=[0 0 0]  TranslationROffset=0  TranslationROffsetUnits=m  TranslationZOffset=0  TranslationZOffsetUnits=m  TranslationThetaOffset=0  TranslationThetaOffsetUnits=deg  RotationMethod=StandardAxis  RotationAngleUnits=deg  RotationStandardAxis=+X  RotationAngle=90  RotationArbitraryAxis=[0 0 1]  FollAlignAxisA=+X  BaseAlignAxisA=+Y  FollAlignAxisB=+Y  BaseAlignAxisB=+Z  RotationSequenceAxes=FollowerAxes  RotationSequence=XYX  RotationSequenceAngles=[0 0 0]  RotationSequenceAnglesUnits=deg  RotationMatrix=[1 0 0; 0 1 0; 0 0 1]
  Transform World2Wall Joint : sm_lib/Frames and Transforms/Rigid Transform  TranslationMethod=Cartesian  TranslationStandardOffset=0.4  TranslationLengthUnit=m  TranslationStandardAxis=+Y  TranslationCartesianOffset=[0 0 0]  TranslationROffset=0  TranslationROffsetUnits=m  TranslationZOffset=0  TranslationZOffsetUnits=m  TranslationThetaOffset=0  TranslationThetaOffsetUnits=deg  RotationMethod=StandardAxis  RotationAngleUnits=deg  RotationStandardAxis=-X  RotationAngle=90  RotationArbitraryAxis=[0 0 1]  FollAlignAxisA=+X  BaseAlignAxisA=+Y  FollAlignAxisB=+Y  BaseAlignAxisB=+Z  RotationSequenceAxes=FollowerAxes  RotationSequence=XYX  RotationSequenceAngles=[0 0 0]  RotationSequenceAnglesUnits=deg  RotationMatrix=[1 0 0; 0 1 0; 0 0 1]
  Wall : Subsystem
  Wall2World : sm_lib/Joints/Prismatic Joint  SenseConstraintForce=off  SenseConstraintForceX=off  SenseConstraintForceY=off  SenseConstraintForceZ=off  SenseConstraintTorque=off  SenseConstraintTorqueX=off  SenseConstraintTorqueY=off  SenseConstraintTorqueZ=off  SenseTotalForce=off  SenseTotalForceX=off  SenseTotalForceY=off  SenseTotalForceZ=off  SenseTotalTorque=off  SenseTotalTorqueX=off  SenseTotalTorqueY=off  SenseTotalTorqueZ=off  CompositeWrenchDir=FollowerOnBase  CompositeWrenchFrame=BaseFrame  EquilibriumPosition=0  EquilibriumPositionUnits=m  SpringStiffness=0  SpringStiffnessUnits=N/m  DampingCoefficient=0  DampingCoefficientUnits=N/(m/s)  TorqueActuationMode=NoTorque  MotionActuationMode=ComputedMotion  SensePosition=off  SenseVelocity=off  SenseAcceleration=off  SenseTorqueForce=off  PositionTargetSpecify=on  PositionTargetPriority=Low  PositionTargetValue=0  PositionTargetValueUnits=m  VelocityTargetSpecify=off  VelocityTargetPriority=High  VelocityTargetValue=0  VelocityTargetValueUnits=m/s
  Ball : PMIOPort  Side=Right
  Ref : PMIOPort  Port=2  Side=Left
  WRf : PMIOPort  Port=3  Side=Left
  CG : PMIOPort  Port=4  Side=Left
  wires:
  2-D Contact Force Circle to Circle/1 -> Terminator/1
  2-D Contact Force Circle to Finite Line/1 -> Terminator1/1
  2-D Contact Force Circle to Circle1/1 -> Terminator2/1
  connections:
  Ref/RConn1 -- Offset and Angle/LConn1
  Wall2World/LConn1 -- Transform Wall2World Joint/RConn1
  Transform World2Wall Joint/LConn1 -- Wall2World/RConn1
  Offset and Angle/RConn1 -- WRf/RConn1 -- Transform World2Wall Joint/RConn1
  Ball/RConn1 -- 2-D Contact Force Circle to Circle1/LConn1 -- 2-D Contact Force Circle to Circle/LConn1 -- 2-D Contact Force Circle to Finite Line/LConn1
  2-D Contact Force Circle to Circle/RConn1 -- Wall/RConn1
  2-D Contact Force Circle to Finite Line/RConn1 -- Wall/RConn2
  Wall/LConn1 -- CG/RConn1 -- Transform Wall2World Joint/LConn1
  2-D Contact Force Circle to Circle1/RConn1 -- Wall/RConn3
